simulink model "CM340A_AdcDiagc"
settings: Solver=FixedStepDiscrete  SolverMode=SingleTasking  StartTime=0.0  StopTime=1  FixedStep=0.002  RelTol=1e-3
values from neighbouring files (symbols this model uses):
  Adc0Diagc = DataDict.NTC    [CM340A_AdcDiagc_DataDict.m]
  Adc1Diagc = DataDict.NTC    [CM340A_AdcDiagc_DataDict.m]
  ADCDIAG0REFVOLT_VOLT_F32 = DataDict.Constant    [CM340A_AdcDiagc_DataDict.m]
  ADCDIAG2REFVOLT_VOLT_F32 = DataDict.Constant    [CM340A_AdcDiagc_DataDict.m]
  ADCDIAG4REFVOLT_VOLT_F32 = DataDict.Constant    [CM340A_AdcDiagc_DataDict.m]
  AdcDiagcNtc0x032FailStep = DataDict.Calibration    [CM340A_AdcDiagc_DataDict.m]
  AdcDiagcNtc0x032PassStep = DataDict.Calibration    [CM340A_AdcDiagc_DataDict.m]
  AdcDiagcNtc0x033FailStep = DataDict.Calibration    [CM340A_AdcDiagc_DataDict.m]
  AdcDiagcNtc0x033PassStep = DataDict.Calibration    [CM340A_AdcDiagc_DataDict.m]
  AdcDiagcSt = DataDict.PIM    [CM340A_AdcDiagc_DataDict.m]
  ADCDIAGPARFLTPRM_CNT_U08 = DataDict.Constant    [CM340A_AdcDiagc_DataDict.m]
  ADCDIAGSCANGROUP2REFFLTPRM_CNT_U08 = DataDict.Constant    [CM340A_AdcDiagc_DataDict.m]
  ADCDIAGSCANGROUP3REFFLTPRM_CNT_U08 = DataDict.Constant    [CM340A_AdcDiagc_DataDict.m]
  ADCDIAGSCANGROUPENDREFVOLT_VOLT_F32 = DataDict.Constant    [CM340A_AdcDiagc_DataDict.m]
  ADCDIAGSCANGROUPSTRTREFVOLT_VOLT_F32 = DataDict.Constant    [CM340A_AdcDiagc_DataDict.m]
  ADCDNECRPARERRCLR_CNT_U08 = DataDict.Constant    [CM340A_AdcDiagc_DataDict.m]
  ADCDNPERPARERRMASK_CNT_U08 = DataDict.Constant    [CM340A_AdcDiagc_DataDict.m]
  VIRTCH21_CNT_U08 = DataDict.Constant    [CM340A_AdcDiagc_DataDict.m]
  VIRTCH22_CNT_U08 = DataDict.Constant    [CM340A_AdcDiagc_DataDict.m]
  VIRTCH23_CNT_U08 = DataDict.Constant    [CM340A_AdcDiagc_DataDict.m]
undefined symbols (not defined in the file or in its folder): NtcSts1, sigbuilder_block, SigQlfr1
libraries: simulink x42, CM340A_AdcDiagc_Library x40
(part 1 of 4)
settings Model: RequirementInfo="{}  %GIDa_ca294f38_ed7c_4fb9_8c54_f4d56271bfc7"  ModifiedHistory=Rev 008: Updated model to Matlab 2013B, added comments to show requirement linkage
settings SolverCC: AutoInsertRateTranBlk=on  InsertRTBMode=Always
settings DataIOCC: SaveFormat=Structure
settings OptimizationCC: BlockReduction=off  InlineParams=on  ZeroExternalMemoryAtStartup=off  ZeroInternalMemoryAtStartup=off  OptimizeModelRefInitCode=on  LifeSpan=1  SimCompilerOptimization=Off
settings DebuggingCC: SignalInfNanChecking=error  SignalRangeChecking=warning  MergeDetectMultiDrivingBlocksExec=none  SolverPrmCheckMsg=error  InheritedTsInSrcMsg=error  DiscreteInheritContinuousMsg=error  SingleTaskRateTransMsg=error  TasksWithSamePriorityMsg=error  SigSpecEnsureSampleTimeMsg=error  CheckMatrixSingularityMsg=error  ParameterUnderflowMsg=error  ParameterPrecisionLossMsg=error  ParameterTunabilityLossMsg=error  FixptConstUnderflowMsg=warning  FixptConstOverflowMsg=warning  VectorMatrixConversionMsg=error  FcnCallInpInsideContextMsg=EnableAllAsError  SignalLabelMismatchMsg=error  UnconnectedInputMsg=error  UnconnectedOutputMsg=error  UnconnectedLineMsg=error  SFcnCompatibilityMsg=error  FrameProcessingCompatibilityMsg=warning  UniqueDataStoreMsg=warning  BusObjectLabelMismatch=error  RootOutportRequireBusObject=error  AssertControl=DisableAll  ModelReferenceIOMsg=error  ModelReferenceVersionMismatchMessage=warning  ModelReferenceIOMismatchMessage=error  ModelReferenceCSMismatchMessage=warning  ModelReferenceDataLoggingMessage=error  StateNameClashWarn=warning  StrictBusMsg=ErrorOnBusTreatedAsVector  NonBusSignalsTreatedAsBus=error  SFInvalidInputDataAccessInChartInitDiag=error  SFTransitionOutsideNaturalParentDiag=error  SFUnconditionalTransitionShadowingDiag=error  SFUndirectedBroadcastEventsDiag=error
settings HardwareCC: ProdBitPerPointer=32  ProdLargestAtomicFloat=None  ProdIntDivRoundTo=Undefined  ProdEndianess=Unspecified  ProdWordSize=32  ProdHWDeviceType=32-bit Generic
settings ModelReferenceCC: ModelReferenceNumInstancesAllowed=Single  PropagateSignalLabelsOutOfModel=off
settings SFSimCC: SimUseLocalCustomCode=off
settings RTWCC: SystemTargetFile=autosar.tlc  GenCodeOnly=on  TemplateMakefile=ert_default_tmf  Description=AUTOSAR  GenerateReport=on  ProcessScript=autosar_make_rtw_hook  RTWUseLocalCustomCode=off  LaunchReport=on  RTWCompilerOptimization=Off
settings CodeAppCC: GenerateComments=off  IgnoreCustomStorageClasses=off  CustomSymbolStrType=$N$R$M  CustomSymbolStrBlkIO=$N$M  SimulinkBlockComments=off
settings STFCustomTargetCC: CodeReplacementLibrary=ANSI_C  ParMdlRefBuildCompliant=on  CompOptLevelCompliant=on  IncludeMdlTerminateFcn=off  CombineOutputUpdateFcns=on  SuppressErrorStatus=on  ERTFirstTimeCompliant=on  ERTCustomFileBanners=on  SupportNonFinite=off  SupportComplex=off  SupportContinuousTime=off  SupportNonInlinedSFcns=off  MATLABClassNameForMDSCustomization=Simulink.SoftwareTarget.ERTCustomization  AutosarCompliant=on  GRTInterface=off  SystemTargetFile=autosar.tlc
settings ERTTargetCC: CodeReplacementLibrary=ANSI_C  MultiwordLength=2048  ConcurrentExecutionCompliant=off  IncludeMdlTerminateFcn=off  SuppressErrorStatus=on  SupportNonFinite=off  SupportComplex=off  ModelStepFunctionPrototypeControlCompliant=off  CPPClassGenCompliant=off  AutosarCompliant=on  InlinedParameterPlacement=NonHierarchical  ERTCustomFileTemplate=example_file_process.tlc  ConvertIfToSwitch=off  SuppressUnreachableDefaultCases=off  EnableUserReplacementTypes=on

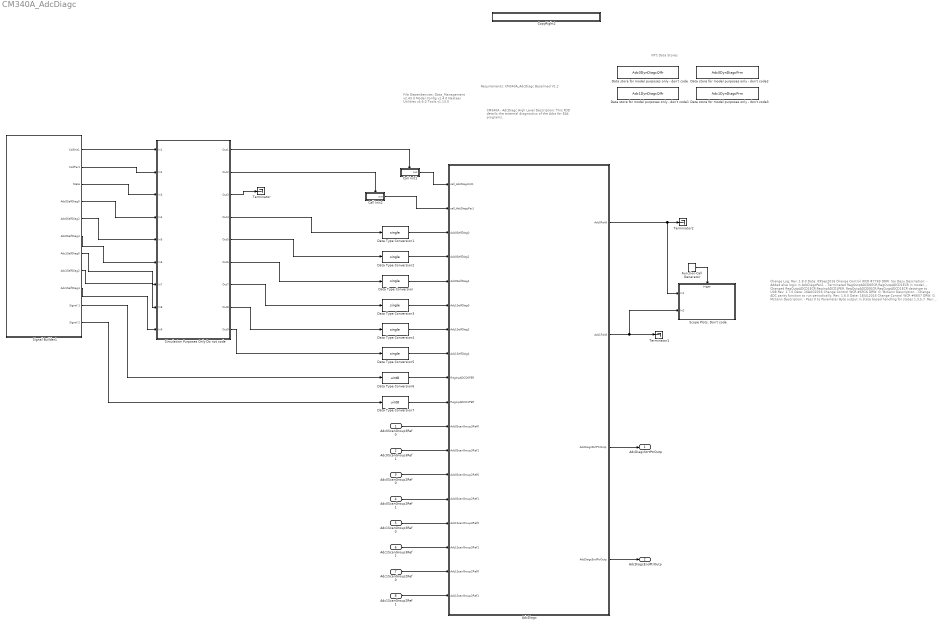
== system CM340A_AdcDiagc ==
  note: NTC Data Stores
  note: CM340A - AdcDiagc
      |
      | High Level Description:
      | This FDD details the external diagnostics of the Adcs for
      | EA4 programs.
  note: Change Log:
      |
      | Rev: 1.8.0
      | Date: 09Sep2016
      | Change Control WCR #7769
      | DRW: Sai Desu
      | Description:
      | - Added else logic in AdcDiagcPer2.
      | - Terminated RegOutpADCD0ECR,RegOutpADCD1ECR in model.
      | - Changed RegOutpADCD1ECR,RegInpADCD1PER, RegOutpADCD0ECR,RegOutpADCD1ECR datatype to U08
      |
      | Rev: 1.7.0
      | Date: 16AUG2016
      | Change Control WCR #6916
      | DRW: G. McCann
      | Description:
      | - Change ADC parity function to run periodically.
      |
      | Rev: 1.6.0
      | Date: 18JUL2016
      | Change Control WCR #6607
      | DRW: G. McCann
      | Description:
      | - Pass 0 to Parameter Byte output in state based handling for states 1,3,5,7.
      |
      | Rev: 1.5.0
      | Date: 15JUL2016
      | Change Control WCR #6588
      | DRW: G. McCann
      | Description:
      | - Change the pass and fail steps for NTCs 0x032 & 0x033 to calibrations instead of config params
      | - Change sequence of state handling in AdcDiagcPer1.  State update should happen last.
      |
      | Rev: 1.4.0
      | Date: 29JUN2016
      | Change Control WCR #6465
      | DRW: G. McCann
      | Description:
      | - Replaced stateflow with equivalent simulink blocks
      | - Requirements linkage added on new blocks
      | - Per1 Adc Diagc Pointer block executes state 6 handling for all cases where Adc Diag State != 0, 2 or 4.  Added
      |   elseif condition for handling of state 6.
      | - Same block needs to send StrtPtr and EndPtr to PIM to hold values between states 0,2,4,6
      | - The StrPtr and EndPtr PIMs should be read to update the outputs from the Adc Daigc Pointer block in Per1.
      |
      | Rev: 1.3.0
      | Date: 22JUN2016
      | Change Control WCR #6418
      | DRW: G. McCann
      | Description:
      | - Remove 'MotCtrl' prefix from I/O not connected to motor control ISR
      |
      | Rev: 1.2.0
      | Date: 07JUN2016
      | Change Control WCR #5774
      | DRW: G. McCann
      | Description:
      | - Change diagnostic parameters on AdcFltCntSt datastores for MIL testing
      | - Change register utilized for parity error check from APDPERRST to ADCDnPER
      | - Change register utilized for parity error clear from APDPERRSTC to ADCDnECR
      | - Add 4 outputs for ADCn start and end pointers (2 per ADC unit).  This change also
      |   eliminates Adc0CfgAndUseAdc0ScanGroup1Cfg and Adc1CfgAndUseAdc1ScanGroup1Cfg
      |   server functions utilized in CM300A and CM320A
      | - Add diagnostics for ADC reference read at the beginning and end of scan groups 2 & 3.  Utilize NTC
      |   Parameter bits 5&6 to accomplish this.
      |
      | Rev: 1.1.0
      | Date: 19MAR2016
      | Change Control WCR #4633,EA4#4637, EA4#4823
      | DRW: Praveen, Muragesh (KPIT)
      | Description:
      | - As per Anomaly CR EA4#3686, the Input Voltage ~= 0  condtion has been changed with
      |  Input Voltage greater than ARCHGLBPRM_FLOATZEROTHD_ULS_F32 in the CM340A_AdcDiagc_Library's
      |  zero check subsystem. ARCHGLBPRM_FLOATZEROTHD_ULS_F32 variable is defined in the .m file.
      |
      | -As per Anomaly CR EA4#3836, SetAdc0ParFlt,SetAdc1ParFlt server runnables have been merged to "SetAdcParFlt".
      | -New inputs 'RegInpAPDPERRST_ADCTL00', 'RegInpAPDPERRST_ADCTL10'
      |  and outputs 'RegOutpAPDPERRSTC_ADCTL00', 'RegOutpAPDPERRSTC_ADCTL10'
      |  and logic related to these has been added
      |
      | - As per Anomaly CR  EA4#4188, fault determination logic has been updated.
      |  8-new PIMs have been created to store fault accumulation avalue in each state for ADC0 and ADC1
      |
      | Rev: 1.0.0
      | Date: 23JAN2014
      | Change Control #: EA4#3400
      | DRW: J. Erlenbeck
      | Description:
      | - Initial Release
      |
      |
      |
      | All changes are highlighted in the red color.
  note: File Dependencies:
      | Data_Management v2.43.0
      | Model Config v1.4.0
      | Nexteer Utilities v4.6.0
      | Tools v1.13.0
  note: Requirements: CM340A_AdcDiagc Baselined V1.2
  Adc0ScanGroup3Ref0 : Inport  RequirementInfo={} %GIDa_49e55e19_ff85_4f6f_a90d_a9dcc2c0ea53
  Adc0ScanGroup3Ref1 : Inport  RequirementInfo={} %GIDa_7dd4fc61_e042_4709_b04f_f275e4d72336  Port=2
  Adc0ScanGroup2Ref0 : Inport  RequirementInfo={} %GIDa_573b7f90_76d7_4d20_8207_3d2b14b10f99  Port=3
  Adc0ScanGroup2Ref1 : Inport  RequirementInfo={} %GIDa_870086a7_d427_43e7_93f7_4a95a875be04  Port=4
  Adc1ScanGroup3Ref0 : Inport  RequirementInfo={} %GIDa_fc4d583e_0d62_4e8f_9497_a2b62302b28b  Port=5
  Adc1ScanGroup3Ref1 : Inport  RequirementInfo={} %GIDa_cad8a16f_cb5f_4c8b_be64_16977f5e4cb9  Port=6
  Adc1ScanGroup2Ref0 : Inport  RequirementInfo={} %GIDa_08b78cad_66ed_443e_a656_dce61b3506e6  Port=7
  Adc1ScanGroup2Ref1 : Inport  RequirementInfo={} %GIDa_f0961ddb_08f8_4c0a_9e27_4a6e0e526bc0  Port=8
  AdcDiagc : Subsystem
  Call Init1 : Subsystem  TreatAsAtomicUnit=on
  Call Init2 : Subsystem  TreatAsAtomicUnit=on
  CopyRight2 : Subsystem  Description=|  mask(Copyright Information){none=on}
      | Copyright info block.                                               
      |                                                                     
      | Place copyright information at the top of every subsystem in design.
      mask prompts: none "No parameters"
      mask help: Place copyright information at the top of every subsystem in design.
      mask Display:
      | NxtrConf = 'Nexteer Confidential';
      | 
      | sys = bdroot; %handle for the current model ("system")
      | first = get_param(sys,'Created');
      | first = first(end-3:end);  %year is last four digits
      | 
      | last = get_param(sys,'LastModifiedDate');
      | if isempty(last)
      |     last = datestr(now,'yyyy');
      | else
      |     last = last(end-3:end);
      | end
      | 
      | if strcmp(first,last)
      |     fprintf('%s -- Copyright %s Nexteer',NxtrConf,first)
      | else
      |     fprintf('%s -- %s%s- %s Nexteer',NxtrConf,char(169),first,last)
      | end
  Data Type Conversion{,1..5} (6 alike) : DataTypeConversion  OutDataTypeStr=single
  Data Type Conversion6 : DataTypeConversion  OutDataTypeStr=uint8
  Data Type Conversion7 : DataTypeConversion  OutDataTypeStr=uint8
  Data store for model purposes only - don't code : DataStoreMemory  DataStoreName=Adc0DynDiagcQlfr
  Data store for model purposes only - don't code1 : DataStoreMemory  DataStoreName=Adc1DynDiagcQlfr
  Data store for model purposes only - don't code2 : DataStoreMemory  DataStoreName=Adc0DynDiagcPrm
  Data store for model purposes only - don't code3 : DataStoreMemory  DataStoreName=Adc1DynDiagcPrm
  Function-Call Generator : simulink/Ports & Subsystems/Function-Call Generator  sample_time=0.002  numberOfIterations=1
  "Scope Plots, Don't code" : Subsystem  TreatAsAtomicUnit=on
  Signal Builder1 : Subsystem  Tag=STV Subsys  LoadFcn=sigbuilder_block('load');  StartFcn=sigbuilder_block('start');  StopFcn=sigbuilder_block('stop');  ClipboardFcn=sigbuilder_block('clipboard');  mask(Sigbuilder block){}
      mask help: Simulink:masks:SigbuilderBlock_MD
      mask init:
      | if ~strcmp(get_param(bdroot(gcbh),'SimulationStatus'),'stopped') tuvar = sigbuilder_block('maskInit'); end
      settings: CopyFcn=sigbuilder_block('copy');  DeleteFcn=sigbuilder_block('delete');  ModelCloseFcn=sigbuilder_block('modelClose');  PreSaveFcn=sigbuilder_block('preSave');  PauseFcn=sigbuilder_block('pause');  ContinueFcn=sigbuilder_block('continue');  NameChangeFcn=sigbuilder_block('namechange');  OpenFcn=sigbuilder_block('open',[88.5 252.75 870.75 494.25 ]);  CloseFcn=sigbuilder_block('close');
      mask Display: plot(0, 0, 100, 100,[2, 2, 32, 32, 2], [68, 8, 8, 68, 68],[32, 2], [38, 38], [32, 19, 2],[53, 60, 44], [32, 17, 17, 2],[16, 16, 31, 31]);txt = getActiveGroup(gcbh);text(2, 100, txt,'verticalAlignment', 'top');
  Simulation Purposes Only Do not code : Subsystem  TreatAsAtomicUnit=on
  Terminator : Terminator
  Terminator1 : Terminator
  Terminator2 : Terminator
  AdcDiagcStrtPtrOutp : Outport
  AdcDiagcEndPtrOutp : Outport  Port=2
  wires:
  Call Init1/1(out) -> AdcDiagc/1(call_AdcDiagcInit1)
  Call Init2/1(out) -> AdcDiagc/2(call_AdcDiagcPer1)
  Data Type Conversion1/1 -> AdcDiagc/3(Adc0SelfDiag0)
  Data Type Conversion2/1 -> AdcDiagc/4(Adc0SelfDiag2)
  Data Type Conversion/1 -> AdcDiagc/5(Adc0SelfDiag4)
  Simulation Purposes Only Do not code/1(Out1) -> Call Init1/Enable
  Simulation Purposes Only Do not code/2(Out2) -> Call Init2/Enable
  Simulation Purposes Only Do not code/4(Out4) -> Data Type Conversion1/1
  Simulation Purposes Only Do not code/5(Out5) -> Data Type Conversion2/1
  Simulation Purposes Only Do not code/6(Out6) -> Data Type Conversion/1
  Simulation Purposes Only Do not code/3(Out3) -> Terminator/1
  Simulation Purposes Only Do not code/7(Out7) -> Data Type Conversion3/1
  Simulation Purposes Only Do not code/8(Out8) -> Data Type Conversion4/1
  Simulation Purposes Only Do not code/9(Out9) -> Data Type Conversion5/1
  Data Type Conversion3/1 -> AdcDiagc/6(Adc1SelfDiag0)
  Data Type Conversion4/1 -> AdcDiagc/7(Adc1SelfDiag2)
  Data Type Conversion5/1 -> AdcDiagc/8(Adc1SelfDiag4)
  AdcDiagc/1(Adc0Faild) -> Terminator2/1, "Scope Plots, Don't code"/1(In1)
  AdcDiagc/2(Adc1Faild) -> Terminator1/1, "Scope Plots, Don't code"/2(In2)
  Signal Builder1/2(CallPer1) -> Simulation Purposes Only Do not code/2(In2)
  Signal Builder1/3(State) -> Simulation Purposes Only Do not code/3(In3)
  Signal Builder1/1(CallInit1) -> Simulation Purposes Only Do not code/1(In1)
  Signal Builder1/8(Adc1SelfDiag2) -> Simulation Purposes Only Do not code/8(In8)
  Signal Builder1/5(Adc0SelfDiag2) -> Simulation Purposes Only Do not code/5(In5)
  Signal Builder1/7(Adc1SelfDiag0) -> Simulation Purposes Only Do not code/7(In7)
  Signal Builder1/4(Adc0SelfDiag0) -> Simulation Purposes Only Do not code/4(In4)
  Signal Builder1/6(Adc0SelfDiag4) -> Simulation Purposes Only Do not code/6(In6)
  Signal Builder1/9(Adc1SelfDiag4) -> Simulation Purposes Only Do not code/9(In9)
  Data Type Conversion6/1 -> AdcDiagc/9(RegInpADCD0PER)
  Data Type Conversion7/1 -> AdcDiagc/10(RegInpADCD1PER)
  AdcDiagc/3(AdcDiagcStrtPtrOutp) -> AdcDiagcStrtPtrOutp/1
  AdcDiagc/4(AdcDiagcEndPtrOutp) -> AdcDiagcEndPtrOutp/1
  Adc0ScanGroup3Ref0/1 -> AdcDiagc/11(Adc0ScanGroup3Ref0)
  Adc0ScanGroup3Ref1/1 -> AdcDiagc/12(Adc0ScanGroup3Ref1)
  Adc0ScanGroup2Ref0/1 -> AdcDiagc/13(Adc0ScanGroup2Ref0)
  Adc0ScanGroup2Ref1/1 -> AdcDiagc/14(Adc0ScanGroup2Ref1)
  Adc1ScanGroup3Ref0/1 -> AdcDiagc/15(Adc1ScanGroup3Ref0)
  Adc1ScanGroup3Ref1/1 -> AdcDiagc/16(Adc1ScanGroup3Ref1)
  Adc1ScanGroup2Ref0/1 -> AdcDiagc/17(Adc1ScanGroup2Ref0)
  Adc1ScanGroup2Ref1/1 -> AdcDiagc/18(Adc1ScanGroup2Ref1)
  Function-Call Generator/1 -> "Scope Plots, Don't code"/Trigger
  Signal Builder1/10(Signal 1) -> Data Type Conversion6/1
  Signal Builder1/11(Signal 2) -> Data Type Conversion7/1

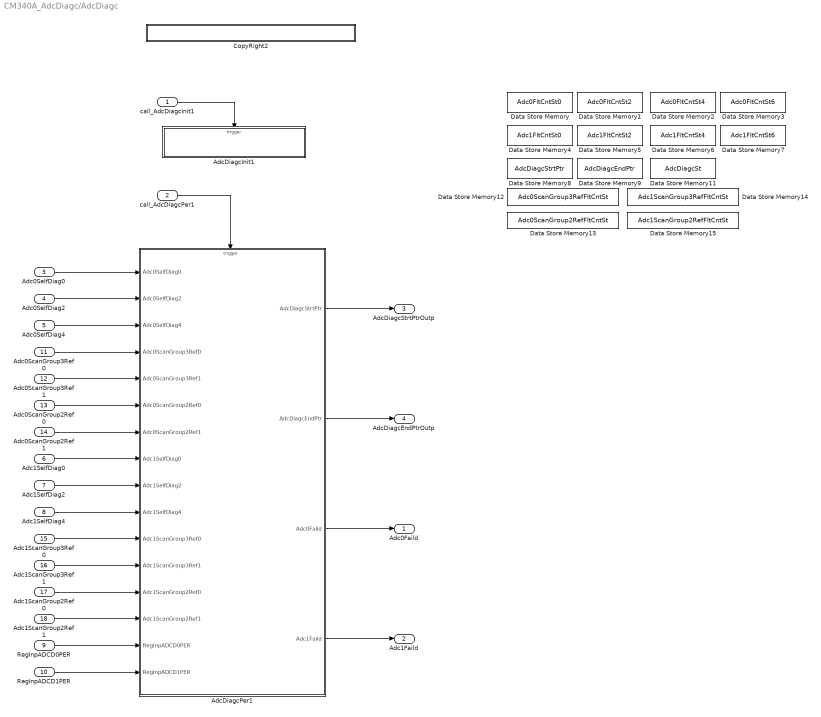
== system CM340A_AdcDiagc/AdcDiagc ==
  call_AdcDiagcInit1 : Inport  RequirementInfo={} %GIDa_18b4b7a7_d8ff_42fd_afd9_8fbc558fb7ae
  call_AdcDiagcPer1 : Inport  RequirementInfo={} %GIDa_8c56c68f_1996_47ee_bda4_35b4dc112bcf  Port=2
  Adc0SelfDiag0 : Inport  RequirementInfo={} %GIDa_768985a4_e900_425c_ae1d_47338650e664  Port=3
  Adc0SelfDiag2 : Inport  RequirementInfo={} %GIDa_3fc10c39_7c74_41d4_a880_daee12f7febc  Port=4
  Adc0SelfDiag4 : Inport  RequirementInfo={} %GIDa_be7414d0_49f3_45cb_bfb1_3ce36dce7edf  Port=5
  Adc1SelfDiag0 : Inport  RequirementInfo={} %GIDa_0acfad8b_9c66_4bcf_95d2_4b0e54aa7e17  Port=6
  Adc1SelfDiag2 : Inport  RequirementInfo={} %GIDa_b99c857a_5fe3_43c9_8cf6_48a3f2428904  Port=7
  Adc1SelfDiag4 : Inport  RequirementInfo={} %GIDa_bb8ad16f_1b31_4872_b9ab_2443b8d4b36b  Port=8
  RegInpADCD0PER : Inport  RequirementInfo={} %GIDa_1c4b2026_055f_43fd_ac9a_1a1cfd812325  Port=9
  RegInpADCD1PER : Inport  RequirementInfo={} %GIDa_ff327575_5ab9_43e4_9182_a2fefb3f953b  Port=10
  Adc0ScanGroup3Ref0 : Inport  RequirementInfo={} %GIDa_bab94f49_6424_4c49_888e_5ff6776a5db3  Port=11
  Adc0ScanGroup3Ref1 : Inport  RequirementInfo={} %GIDa_98f92e48_b093_40f2_8328_2158e7be4df2  Port=12
  Adc0ScanGroup2Ref0 : Inport  RequirementInfo={} %GIDa_ab2ebf3d_54de_4695_942c_c5c65492a51c  Port=13
  Adc0ScanGroup2Ref1 : Inport  RequirementInfo={} %GIDa_8b71ec07_3ef8_4676_a6fa_bdb7f3897266  Port=14
  Adc1ScanGroup3Ref0 : Inport  RequirementInfo={} %GIDa_572c4384_6519_48a1_aa24_069bc074be5f  Port=15
  Adc1ScanGroup3Ref1 : Inport  RequirementInfo={} %GIDa_259d8fd0_61d2_4bba_b7a5_11056a435558  Port=16
  Adc1ScanGroup2Ref0 : Inport  RequirementInfo={} %GIDa_18152ad2_e8f7_4af5_a23a_ab069d03dc39  Port=17
  Adc1ScanGroup2Ref1 : Inport  RequirementInfo={} %GIDa_93789243_a541_499f_9474_e657f20cd06a  Port=18
  AdcDiagcInit1 : Subsystem
  AdcDiagcPer1 : Subsystem  RequirementInfo="{'linktype_rmi_doors' '000079f2 (/ESG Group/FDD Module Requirements/EA4 Specific/CM340A_AdcDiagc)' '#CM340A_16' 'true' 'REQ:  CM340A_16' '' ; 'linktype_rmi_doors' '000079f2 (/ESG Group/FDD Module Requirements/EA4 Specific/CM340A_AdcDiagc)' '#CM340A_70' 'true' 'REQ:  CM340A_70' '' ; 'linktype_rmi_doors' '000079f2 (/ESG Group/FDD Module Requirements/EA4 Specific/CM340A_AdcDiagc)' '#CM340A_204' 'true' 'REQ:  CM340A_204' '' } %GIDa_212d137a_62a0_40b8_86f5_bba5fab12a7f"  TreatAsAtomicUnit=on
  CopyRight2 : Subsystem  Description=|  mask(Copyright Information){none=on}
      | Copyright info block.                                               
      |                                                                     
      | Place copyright information at the top of every subsystem in design.
      mask prompts: none "No parameters"
      mask help: Place copyright information at the top of every subsystem in design.
      mask Display:
      | NxtrConf = 'Nexteer Confidential';
      | 
      | sys = bdroot; %handle for the current model ("system")
      | first = get_param(sys,'Created');
      | first = first(end-3:end);  %year is last four digits
      | 
      | last = get_param(sys,'LastModifiedDate');
      | if isempty(last)
      |     last = datestr(now,'yyyy');
      | else
      |     last = last(end-3:end);
      | end
      | 
      | if strcmp(first,last)
      |     fprintf('%s -- Copyright %s Nexteer',NxtrConf,first)
      | else
      |     fprintf('%s -- %s%s- %s Nexteer',NxtrConf,char(169),first,last)
      | end
  Data Store Memory : DataStoreMemory  DataStoreName=Adc0FltCntSt0  StateMustResolveToSignalObject=on
  Data Store Memory1 : DataStoreMemory  DataStoreName=Adc0FltCntSt2  StateMustResolveToSignalObject=on
  Data Store Memory11 : DataStoreMemory  DataStoreName=AdcDiagcSt  StateMustResolveToSignalObject=on
  Data Store Memory12 : DataStoreMemory  DataStoreName=Adc0ScanGroup3RefFltCntSt  StateMustResolveToSignalObject=on
  Data Store Memory13 : DataStoreMemory  DataStoreName=Adc0ScanGroup2RefFltCntSt  StateMustResolveToSignalObject=on
  Data Store Memory14 : DataStoreMemory  DataStoreName=Adc1ScanGroup3RefFltCntSt  StateMustResolveToSignalObject=on
  Data Store Memory15 : DataStoreMemory  DataStoreName=Adc1ScanGroup2RefFltCntSt  StateMustResolveToSignalObject=on
  Data Store Memory2 : DataStoreMemory  DataStoreName=Adc0FltCntSt4  StateMustResolveToSignalObject=on
  Data Store Memory3 : DataStoreMemory  DataStoreName=Adc0FltCntSt6  StateMustResolveToSignalObject=on
  Data Store Memory4 : DataStoreMemory  DataStoreName=Adc1FltCntSt0  StateMustResolveToSignalObject=on
  Data Store Memory5 : DataStoreMemory  DataStoreName=Adc1FltCntSt2  StateMustResolveToSignalObject=on
  Data Store Memory6 : DataStoreMemory  DataStoreName=Adc1FltCntSt4  StateMustResolveToSignalObject=on
  Data Store Memory7 : DataStoreMemory  DataStoreName=Adc1FltCntSt6  StateMustResolveToSignalObject=on
  Data Store Memory8 : DataStoreMemory  DataStoreName=AdcDiagcStrtPtr  StateMustResolveToSignalObject=on
  Data Store Memory9 : DataStoreMemory  DataStoreName=AdcDiagcEndPtr  StateMustResolveToSignalObject=on
  Adc0Faild : Outport
  Adc1Faild : Outport  Port=2
  AdcDiagcStrtPtrOutp : Outport  Port=3
  AdcDiagcEndPtrOutp : Outport  Port=4
  wires:
  call_AdcDiagcInit1/1 -> AdcDiagcInit1/Trigger
  call_AdcDiagcPer1/1 -> AdcDiagcPer1/Trigger
  Adc0SelfDiag0/1 -> AdcDiagcPer1/1(Adc0SelfDiag0)
  Adc0SelfDiag2/1 -> AdcDiagcPer1/2(Adc0SelfDiag2)
  Adc0SelfDiag4/1 -> AdcDiagcPer1/3(Adc0SelfDiag4)
  Adc1SelfDiag0/1 -> AdcDiagcPer1/8(Adc1SelfDiag0)
  Adc1SelfDiag2/1 -> AdcDiagcPer1/9(Adc1SelfDiag2)
  Adc1SelfDiag4/1 -> AdcDiagcPer1/10(Adc1SelfDiag4)
  Adc0ScanGroup3Ref0/1 -> AdcDiagcPer1/4(Adc0ScanGroup3Ref0)
  Adc0ScanGroup3Ref1/1 -> AdcDiagcPer1/5(Adc0ScanGroup3Ref1)
  Adc0ScanGroup2Ref0/1 -> AdcDiagcPer1/6(Adc0ScanGroup2Ref0)
  Adc0ScanGroup2Ref1/1 -> AdcDiagcPer1/7(Adc0ScanGroup2Ref1)
  Adc1ScanGroup3Ref0/1 -> AdcDiagcPer1/11(Adc1ScanGroup3Ref0)
  Adc1ScanGroup3Ref1/1 -> AdcDiagcPer1/12(Adc1ScanGroup3Ref1)
  Adc1ScanGroup2Ref0/1 -> AdcDiagcPer1/13(Adc1ScanGroup2Ref0)
  Adc1ScanGroup2Ref1/1 -> AdcDiagcPer1/14(Adc1ScanGroup2Ref1)
  AdcDiagcPer1/1(AdcDiagcStrtPtr) -> AdcDiagcStrtPtrOutp/1
  AdcDiagcPer1/2(AdcDiagcEndPtr) -> AdcDiagcEndPtrOutp/1
  RegInpADCD0PER/1 -> AdcDiagcPer1/15(RegInpADCD0PER)
  RegInpADCD1PER/1 -> AdcDiagcPer1/16(RegInpADCD1PER)
  AdcDiagcPer1/3(Adc0Faild) -> Adc0Faild/1
  AdcDiagcPer1/4(Adc1Faild) -> Adc1Faild/1

== system CM340A_AdcDiagc/Call Init1 ==
  Enable : EnablePort
  Function Call Trigger : simulink/Ports & Subsystems/Function-Call Generator  RequirementInfo={} %GIDa_ff755a2e_49d1_45f7_8591_3ce0ef475338  sample_time=0.002  numberOfIterations=1
  out : Outport
  wires:
  Function Call Trigger/1 -> out/1

== system CM340A_AdcDiagc/Call Init2 ==
  Enable : EnablePort
  Function Call Trigger : simulink/Ports & Subsystems/Function-Call Generator  RequirementInfo={} %GIDa_6dd05ab1_f91b_4d7a_a0ec_1170d213fa7b  sample_time=0.002  numberOfIterations=1
  out : Outport
  wires:
  Function Call Trigger/1 -> out/1

== system CM340A_AdcDiagc/CopyRight2 ==

== system CM340A_AdcDiagc/Scope Plots, Don't code ==
  In1 : Inport
  In2 : Inport  Port=2
  function : TriggerPort  TriggerType=function-call
  Data Store Read : DataStoreRead  DataStoreName=Adc0DynDiagcPrm
  Data Store Read1 : DataStoreRead  DataStoreName=Adc1DynDiagcPrm
  Display : Display
  Display1 : Display
  Scope : Scope  NumInputPorts=4
      settings: YMin=-5~-5~-5~-5  YMax=5~5~5~5
  wires:
  Data Store Read/1 -> Display/1, Scope/2
  Data Store Read1/1 -> Display1/1, Scope/4
  In1/1 -> Scope/1
  In2/1 -> Scope/3

== system CM340A_AdcDiagc/Signal Builder1 ==
  Demux : Demux  Tag=STV Demux  Outputs=11
  FromWs : FromWorkspace  Tag=STV FromWs  VariableName=tuvar  SampleTime=0
  CallInit1 : Outport
  CallPer1 : Outport  Tag=STV Outport  Port=2
  State : Outport  Tag=STV Outport  Port=3
  Adc0SelfDiag0 : Outport  Tag=STV Outport  Port=4
  Adc0SelfDiag2 : Outport  Tag=STV Outport  Port=5
  Adc0SelfDiag4 : Outport  Tag=STV Outport  Port=6
  Adc1SelfDiag0 : Outport  Tag=STV Outport  Port=7
  Adc1SelfDiag2 : Outport  Tag=STV Outport  Port=8
  Adc1SelfDiag4 : Outport  Tag=STV Outport  Port=9
  Signal 1 : Outport  Tag=STV Outport  Port=10
  Signal 2 : Outport  Tag=STV Outport  Port=11
  wires:
  Demux/1 -> CallInit1/1
  FromWs/1 -> Demux/1
  Demux/2 -> CallPer1/1
  Demux/3 -> State/1
  Demux/4 -> Adc0SelfDiag0/1
  Demux/5 -> Adc0SelfDiag2/1
  Demux/6 -> Adc0SelfDiag4/1
  Demux/7 -> Adc1SelfDiag0/1
  Demux/8 -> Adc1SelfDiag2/1
  Demux/9 -> Adc1SelfDiag4/1
  Demux/10 -> Signal 1/1
  Demux/11 -> Signal 2/1

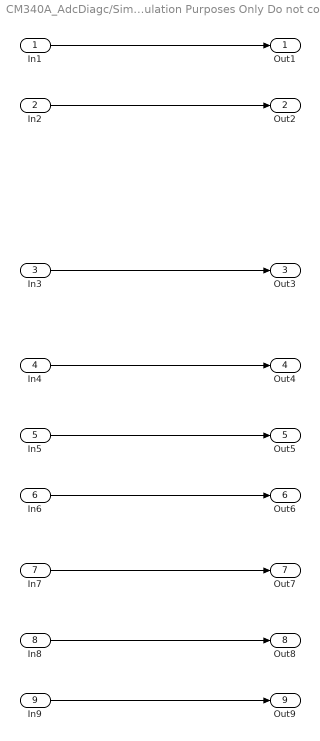
== system CM340A_AdcDiagc/Simulation Purposes Only Do not code ==
  In1 : Inport
  In2 : Inport  Port=2
  In3 : Inport  Port=3
  In4 : Inport  Port=4
  In5 : Inport  Port=5
  In6 : Inport  Port=6
  In7 : Inport  Port=7
  In8 : Inport  Port=8
  In9 : Inport  Port=9
  Out1 : Outport
  Out2 : Outport  Port=2
  Out3 : Outport  Port=3
  Out4 : Outport  Port=4
  Out5 : Outport  Port=5
  Out6 : Outport  Port=6
  Out7 : Outport  Port=7
  Out8 : Outport  Port=8
  Out9 : Outport  Port=9
  wires:
  In1/1 -> Out1/1
  In2/1 -> Out2/1
  In3/1 -> Out3/1
  In4/1 -> Out4/1
  In5/1 -> Out5/1
  In6/1 -> Out6/1
  In7/1 -> Out7/1
  In8/1 -> Out8/1
  In9/1 -> Out9/1

== system CM340A_AdcDiagc/AdcDiagc/AdcDiagcInit1 ==
  function : TriggerPort  TriggerType=function-call
  CopyRight2 : Subsystem  Description=|  mask(Copyright Information){none=on}
      | Copyright info block.                                               
      |                                                                     
      | Place copyright information at the top of every subsystem in design.
      mask prompts: none "No parameters"
      mask help: Place copyright information at the top of every subsystem in design.
      mask Display:
      | NxtrConf = 'Nexteer Confidential';
      | 
      | sys = bdroot; %handle for the current model ("system")
      | first = get_param(sys,'Created');
      | first = first(end-3:end);  %year is last four digits
      | 
      | last = get_param(sys,'LastModifiedDate');
      | if isempty(last)
      |     last = datestr(now,'yyyy');
      | else
      |     last = last(end-3:end);
      | end
      | 
      | if strcmp(first,last)
      |     fprintf('%s -- Copyright %s Nexteer',NxtrConf,first)
      | else
      |     fprintf('%s -- %s%s- %s Nexteer',NxtrConf,char(169),first,last)
      | end

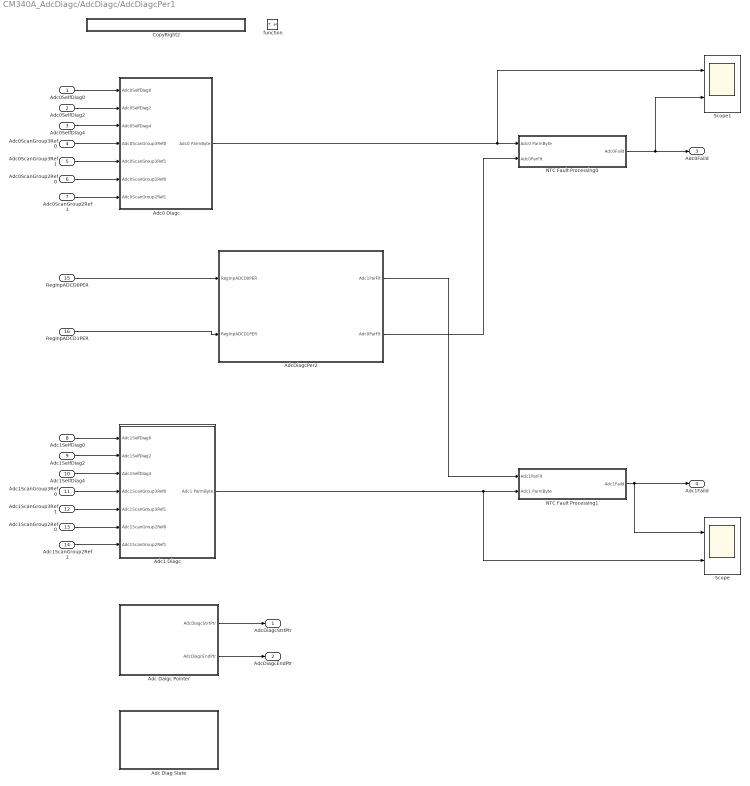
== system CM340A_AdcDiagc/AdcDiagc/AdcDiagcPer1 ==
  Adc0SelfDiag0 : Inport  RequirementInfo={} %GIDa_398af57d_66f9_4248_8190_db0e776b721c
  Adc0SelfDiag2 : Inport  RequirementInfo={} %GIDa_3797a2ee_2714_4505_8d9f_c06ba9c2410a  Port=2
  Adc0SelfDiag4 : Inport  RequirementInfo={} %GIDa_1ba69c54_a3c2_4a1b_b281_43e29c60c561  Port=3
  Adc0ScanGroup3Ref0 : Inport  RequirementInfo={} %GIDa_b69125fd_1372_4953_9f1d_8e09c2ad4765  Port=4
  Adc0ScanGroup3Ref1 : Inport  RequirementInfo={} %GIDa_f2d9eb47_94c7_42c7_a565_8454874220f9  Port=5
  Adc0ScanGroup2Ref0 : Inport  RequirementInfo={} %GIDa_748996a5_f302_4c6d_9251_b06a31b520da  Port=6
  Adc0ScanGroup2Ref1 : Inport  RequirementInfo={} %GIDa_62cd2350_592e_4caf_8293_5786819e876e  Port=7
  Adc1SelfDiag0 : Inport  RequirementInfo={} %GIDa_5433d538_46b8_4710_9f51_90a1755e5365  Port=8
  Adc1SelfDiag2 : Inport  RequirementInfo={} %GIDa_cf98083c_832e_42bb_b714_4f1778ae5820  Port=9
  Adc1SelfDiag4 : Inport  RequirementInfo={} %GIDa_f0469ca3_52bb_4d75_9ba6_24b9dcc42878  Port=10
  Adc1ScanGroup3Ref0 : Inport  RequirementInfo={} %GIDa_8fb83cb2_3080_4b0a_be49_1e0ee5149889  Port=11
  Adc1ScanGroup3Ref1 : Inport  RequirementInfo={} %GIDa_9cfb09be_3cef_48c6_a43d_b09581d94508  Port=12
  Adc1ScanGroup2Ref0 : Inport  RequirementInfo={} %GIDa_19dd82f8_e08f_4772_9f75_eda53b43109c  Port=13
  Adc1ScanGroup2Ref1 : Inport  RequirementInfo={} %GIDa_5081205f_adca_4d34_ac0d_2760b9b6cbb4  Port=14
  RegInpADCD0PER : Inport  RequirementInfo={} %GIDa_f892c6be_11e8_41e7_9539_6ea24d7285ca  Port=15
  RegInpADCD1PER : Inport  RequirementInfo={} %GIDa_fb1af02a_ee48_4694_a668_6f65c74c073f  Port=16
  function : TriggerPort  TriggerType=function-call
  Adc Daigc Pointer : Subsystem  Priority=20
      settings: AttributesFormatString=Priority=%<Priority>
  Adc Diag State : Subsystem  RequirementInfo="{'linktype_rmi_doors' '000079f2 (/ESG Group/FDD Module Requirements/EA4 Specific/CM340A_AdcDiagc)' '#CM340A_194' 'true' 'REQ:  CM340A_194' '' ; 'linktype_rmi_doors' '000079f2 (/ESG Group/FDD Module Requirements/EA4 Specific/CM340A_AdcDiagc)' '#CM340A_102' 'true' 'REQ:  CM340A_102' '' ; 'linktype_rmi_doors' '000079f2 (/ESG Group/FDD Module Requirements/EA4 Specific/CM340A_AdcDiagc)' '#CM340A_112' 'true' 'REQ:  CM340A_112' '' } %GIDa_801c7126_d3ff_4755_b335_51df2b5f807d"  Priority=40  TreatAsAtomicUnit=on
      settings: AttributesFormatString=Priority = %<Priority>
  Adc0 Diagc : Subsystem  Priority=5  TreatAsAtomicUnit=on
      settings: AttributesFormatString=Priority=%<Priority>
  Adc1 Diagc : Subsystem  Priority=10  TreatAsAtomicUnit=on
      settings: AttributesFormatString=Priority=%<Priority>
  AdcDiagcPer2 : Subsystem  RequirementInfo="{'linktype_rmi_doors' '000079f2 (/ESG Group/FDD Module Requirements/EA4 Specific/CM340A_AdcDiagc)' '#CM340A_206' 'true' 'REQ:  CM340A_206' '' } %GIDa_5b7560d5_8186_4135_8b2d_fba8c958e2d9"  Priority=0
      settings: AttributesFormatString=Priority = %<Priority>
  CopyRight2 : Subsystem  Description=|  mask(Copyright Information){none=on}
      | Copyright info block.                                               
      |                                                                     
      | Place copyright information at the top of every subsystem in design.
      mask prompts: none "No parameters"
      mask help: Place copyright information at the top of every subsystem in design.
      mask Display:
      | NxtrConf = 'Nexteer Confidential';
      | 
      | sys = bdroot; %handle for the current model ("system")
      | first = get_param(sys,'Created');
      | first = first(end-3:end);  %year is last four digits
      | 
      | last = get_param(sys,'LastModifiedDate');
      | if isempty(last)
      |     last = datestr(now,'yyyy');
      | else
      |     last = last(end-3:end);
      | end
      | 
      | if strcmp(first,last)
      |     fprintf('%s -- Copyright %s Nexteer',NxtrConf,first)
      | else
      |     fprintf('%s -- %s%s- %s Nexteer',NxtrConf,char(169),first,last)
      | end
  NTC Fault Processing0 : Subsystem  RequirementInfo="{'linktype_rmi_doors' '000079f2 (/ESG Group/FDD Module Requirements/EA4 Specific/CM340A_AdcDiagc)' '#CM340A_200' 'true' 'REQ:  CM340A_200' '' ; 'linktype_rmi_doors' '000079f2 (/ESG Group/FDD Module Requirements/EA4 Specific/CM340A_AdcDiagc)' '#CM340A_122' 'true' 'REQ:  CM340A_122' '' } %GIDa_4d05836e_001f_46e0_8cc5_082fda3c5ac5"  TreatAsAtomicUnit=on
  NTC Fault Processing1 : Subsystem  RequirementInfo="{'linktype_rmi_doors' '000079f2 (/ESG Group/FDD Module Requirements/EA4 Specific/CM340A_AdcDiagc)' '#CM340A_203' 'true' 'REQ:  CM340A_203' '' ; 'linktype_rmi_doors' '000079f2 (/ESG Group/FDD Module Requirements/EA4 Specific/CM340A_AdcDiagc)' '#CM340A_132' 'true' 'REQ:  CM340A_132' '' } %GIDa_2135f153_303a_4bc7_a24b_680511b64853"  TreatAsAtomicUnit=on
  Scope : Scope  NumInputPorts=2
      settings: YMin=-5~-5  YMax=5~5
  Scope1 : Scope  NumInputPorts=2
      settings: YMin=-5~-5  YMax=5~5  SaveName=ScopeData9
  AdcDiagcStrtPtr : Outport
  AdcDiagcEndPtr : Outport  Port=2
  Adc0Faild : Outport  Port=3
  Adc1Faild : Outport  Port=4
  wires:
  Adc1SelfDiag0/1 -> Adc1 Diagc/1(Adc1SelfDiag0)
  Adc1SelfDiag2/1 -> Adc1 Diagc/2(Adc1SelfDiag2)
  Adc1SelfDiag4/1 -> Adc1 Diagc/3(Adc1SelfDiag4)
  Adc0SelfDiag0/1 -> Adc0 Diagc/1(Adc0SelfDiag0)
  Adc0SelfDiag2/1 -> Adc0 Diagc/2(Adc0SelfDiag2)
  Adc0SelfDiag4/1 -> Adc0 Diagc/3(Adc0SelfDiag4)
  Adc0ScanGroup3Ref0/1 -> Adc0 Diagc/4(Adc0ScanGroup3Ref0)
  Adc0ScanGroup3Ref1/1 -> Adc0 Diagc/5(Adc0ScanGroup3Ref1)
  Adc0ScanGroup2Ref0/1 -> Adc0 Diagc/6(Adc0ScanGroup2Ref0)
  Adc0ScanGroup2Ref1/1 -> Adc0 Diagc/7(Adc0ScanGroup2Ref1)
  Adc1ScanGroup3Ref0/1 -> Adc1 Diagc/4(Adc1ScanGroup3Ref0)
  Adc1ScanGroup3Ref1/1 -> Adc1 Diagc/5(Adc1ScanGroup3Ref1)
  Adc1ScanGroup2Ref0/1 -> Adc1 Diagc/6(Adc1ScanGroup2Ref0)
  Adc1ScanGroup2Ref1/1 -> Adc1 Diagc/7(Adc1ScanGroup2Ref1)
  Adc Daigc Pointer/1(AdcDiagcStrtPtr) -> AdcDiagcStrtPtr/1
  Adc Daigc Pointer/2(AdcDiagcEndPtr) -> AdcDiagcEndPtr/1
  RegInpADCD0PER/1 -> AdcDiagcPer2/1(RegInpADCD0PER)
  RegInpADCD1PER/1 -> AdcDiagcPer2/2(RegInpADCD1PER)
  NTC Fault Processing0/1(Adc0Faild) -> Scope1/2, Adc0Faild/1
  Adc0 Diagc/1(Adc0 ParmByte) -> Scope1/1, NTC Fault Processing0/1(Adc0 ParmByte)
  NTC Fault Processing1/1(Adc1Faild) -> Scope/1, Adc1Faild/1
  Adc1 Diagc/1(Adc1 ParmByte) -> Scope/2, NTC Fault Processing1/2(Adc1 ParmByte)
  AdcDiagcPer2/2(Adc0ParFlt) -> NTC Fault Processing0/2(Adc0ParFlt)
  AdcDiagcPer2/1(Adc1ParFlt) -> NTC Fault Processing1/1(Adc1ParFlt)

== system CM340A_AdcDiagc/AdcDiagc/CopyRight2 ==

== system CM340A_AdcDiagc/AdcDiagc/AdcDiagcInit1/CopyRight2 ==

== system CM340A_AdcDiagc/AdcDiagc/AdcDiagcPer1/Adc Daigc Pointer ==
  CopyRight2 : Subsystem  Description=|  mask(Copyright Information){none=on}
      | Copyright info block.                                               
      |                                                                     
      | Place copyright information at the top of every subsystem in design.
      mask prompts: none "No parameters"
      mask help: Place copyright information at the top of every subsystem in design.
      mask Display:
      | NxtrConf = 'Nexteer Confidential';
      | 
      | sys = bdroot; %handle for the current model ("system")
      | first = get_param(sys,'Created');
      | first = first(end-3:end);  %year is last four digits
      | 
      | last = get_param(sys,'LastModifiedDate');
      | if isempty(last)
      |     last = datestr(now,'yyyy');
      | else
      |     last = last(end-3:end);
      | end
      | 
      | if strcmp(first,last)
      |     fprintf('%s -- Copyright %s Nexteer',NxtrConf,first)
      | else
      |     fprintf('%s -- %s%s- %s Nexteer',NxtrConf,char(169),first,last)
      | end
  Data Store Read : DataStoreRead  DataStoreName=AdcDiagcSt
  Strt & End Ptr Output : Subsystem  Priority=2
      settings: AttributesFormatString=Priority = %<Priority>
  Strt & End Ptr Store : Subsystem  Priority=1
      settings: AttributesFormatString=Priority = %<Priority>
  AdcDiagcStrtPtr : Outport
  AdcDiagcEndPtr : Outport  Port=2
  wires:
  Data Store Read/1 -> Strt & End Ptr Store/1(Adc Diag State)
  Strt & End Ptr Output/1(AdcDiagcStrtPtr) -> AdcDiagcStrtPtr/1
  Strt & End Ptr Output/2(AdcDiagcEndPtr) -> AdcDiagcEndPtr/1

== system CM340A_AdcDiagc/AdcDiagc/AdcDiagcPer1/Adc Diag State ==
  note: ***********************************************
      | Note that this mechanism of
      | rolling back the state to 0 with this
      | method only works when
      | AdcDiagcSt.EngMax = 7.  If the diagnostic
      | changes this technique will have to be revisted
      | ***********************************************
  Add : Sum
  Bitwise Operator : simulink/Logic and Bit Operations/Bitwise Operator  logicop=AND  UseBitMask=off  NumInputPorts=2  BitMask=bin2dec('11011001')  BitMaskRealWorld=Stored Integer
  Constant : Constant  OutDataTypeStr=uint8
  Constant1 : Constant  Value=AdcDiagcSt.EngMax
  CopyRight2 : Subsystem  Description=|  mask(Copyright Information){none=on}
      | Copyright info block.                                               
      |                                                                     
      | Place copyright information at the top of every subsystem in design.
      mask prompts: none "No parameters"
      mask help: Place copyright information at the top of every subsystem in design.
      mask Display:
      | NxtrConf = 'Nexteer Confidential';
      | 
      | sys = bdroot; %handle for the current model ("system")
      | first = get_param(sys,'Created');
      | first = first(end-3:end);  %year is last four digits
      | 
      | last = get_param(sys,'LastModifiedDate');
      | if isempty(last)
      |     last = datestr(now,'yyyy');
      | else
      |     last = last(end-3:end);
      | end
      | 
      | if strcmp(first,last)
      |     fprintf('%s -- Copyright %s Nexteer',NxtrConf,first)
      | else
      |     fprintf('%s -- %s%s- %s Nexteer',NxtrConf,char(169),first,last)
      | end
  Data Store Read : DataStoreRead  DataStoreName=AdcDiagcSt
  Data Store Write : DataStoreWrite  DataStoreName=AdcDiagcSt
  Data Type Conversion : DataTypeConversion  OutDataTypeStr=uint8
  wires:
  Constant/1 -> Add/1
  Constant1/1 -> Data Type Conversion/1
  Add/1 -> Bitwise Operator/2
  Data Type Conversion/1 -> Bitwise Operator/1
  Data Store Read/1 -> Add/2
  Bitwise Operator/1 -> Data Store Write/1

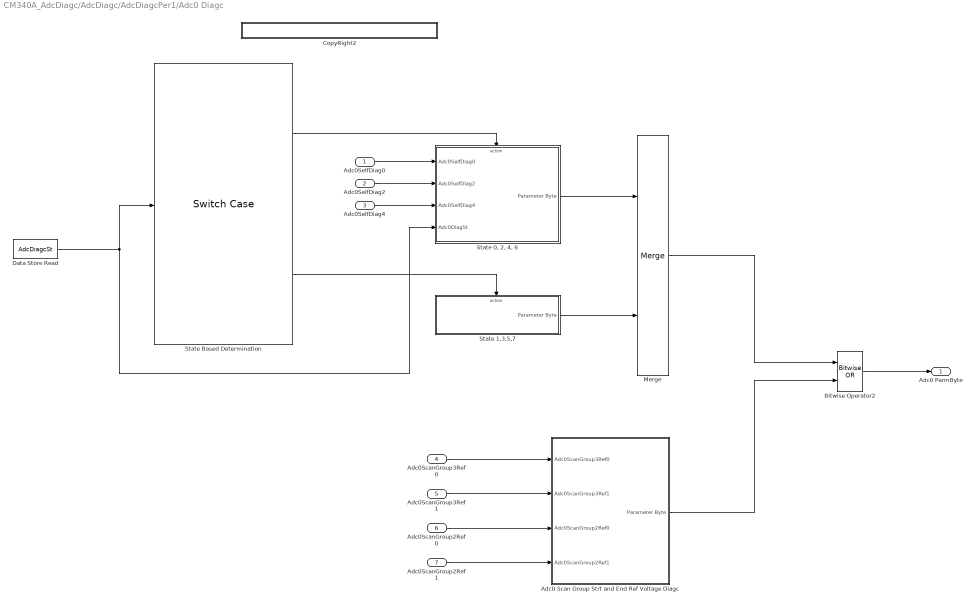
== system CM340A_AdcDiagc/AdcDiagc/AdcDiagcPer1/Adc0 Diagc ==
  Adc0SelfDiag0 : Inport  RequirementInfo={} %GIDa_8c44b7b5_be32_46ad_bd4e_9c60b23c45a8
  Adc0SelfDiag2 : Inport  RequirementInfo={} %GIDa_a296aa7a_0e47_453a_a758_f77e1172a5a6  Port=2
  Adc0SelfDiag4 : Inport  RequirementInfo={} %GIDa_a98d8dd3_9f46_4309_b7f1_a50f146190a2  Port=3
  Adc0ScanGroup3Ref0 : Inport  RequirementInfo={} %GIDa_11954da4_53ef_4f14_b015_a9bd1937ba50  Port=4
  Adc0ScanGroup3Ref1 : Inport  RequirementInfo={} %GIDa_778518f3_3d70_4d5f_997f_17df4302258d  Port=5
  Adc0ScanGroup2Ref0 : Inport  RequirementInfo={} %GIDa_4d51d9ac_68cd_474e_b511_5bbbc9264d7b  Port=6
  Adc0ScanGroup2Ref1 : Inport  RequirementInfo={} %GIDa_f8618099_7dc5_498a_97eb_bfbda85dffb1  Port=7
  Adc0 Scan Group Strt and End Ref Voltage Diagc : Subsystem  RequirementInfo="{'linktype_rmi_doors' '000079f2 (/ESG Group/FDD Module Requirements/EA4 Specific/CM340A_AdcDiagc)' '#CM340A_204' 'true' 'REQ:  CM340A_204' '' } %GIDa_42a8a50a_2387_4959_8004_357af6557f2b"  Priority=20
      settings: AttributesFormatString=Priority = %<Priority>
  Bitwise Operator2 : simulink/Logic and Bit Operations/Bitwise Operator  logicop=OR  UseBitMask=off  NumInputPorts=2  BitMask=bin2dec('11011001')  BitMaskRealWorld=Stored Integer
  CopyRight2 : Subsystem  Description=|  mask(Copyright Information){none=on}
      | Copyright info block.                                               
      |                                                                     
      | Place copyright information at the top of every subsystem in design.
      mask prompts: none "No parameters"
      mask help: Place copyright information at the top of every subsystem in design.
      mask Display:
      | NxtrConf = 'Nexteer Confidential';
      | 
      | sys = bdroot; %handle for the current model ("system")
      | first = get_param(sys,'Created');
      | first = first(end-3:end);  %year is last four digits
      | 
      | last = get_param(sys,'LastModifiedDate');
      | if isempty(last)
      |     last = datestr(now,'yyyy');
      | else
      |     last = last(end-3:end);
      | end
      | 
      | if strcmp(first,last)
      |     fprintf('%s -- Copyright %s Nexteer',NxtrConf,first)
      | else
      |     fprintf('%s -- %s%s- %s Nexteer',NxtrConf,char(169),first,last)
      | end
  Data Store Read : DataStoreRead  DataStoreName=AdcDiagcSt
  Merge : Merge
  "State 0, 2, 4, 6" : Subsystem  TreatAsAtomicUnit=on
  State 1,3,5,7 : Subsystem  TreatAsAtomicUnit=on
  State Based Determination : SwitchCase  CaseConditions={[0,2,4,6]}
  Adc0 ParmByte : Outport
  wires:
  Adc0SelfDiag0/1 -> "State 0, 2, 4, 6"/1(Adc0SelfDiag0)
  Adc0SelfDiag2/1 -> "State 0, 2, 4, 6"/2(Adc0SelfDiag2)
  Adc0SelfDiag4/1 -> "State 0, 2, 4, 6"/3(Adc0SelfDiag4)
  Data Store Read/1 -> "State 0, 2, 4, 6"/4(Adc0DiagSt), State Based Determination/1
  State Based Determination/1 -> "State 0, 2, 4, 6"/Action
  State Based Determination/2 -> State 1,3,5,7/Action
  Adc0ScanGroup3Ref0/1 -> Adc0 Scan Group Strt and End Ref Voltage Diagc/1(Adc0ScanGroup3Ref0)
  Adc0ScanGroup3Ref1/1 -> Adc0 Scan Group Strt and End Ref Voltage Diagc/2(Adc0ScanGroup3Ref1)
  Adc0ScanGroup2Ref0/1 -> Adc0 Scan Group Strt and End Ref Voltage Diagc/3(Adc0ScanGroup2Ref0)
  Adc0ScanGroup2Ref1/1 -> Adc0 Scan Group Strt and End Ref Voltage Diagc/4(Adc0ScanGroup2Ref1)
  "State 0, 2, 4, 6"/1(Parameter Byte) -> Merge/1
  State 1,3,5,7/1(Parameter Byte) -> Merge/2
  Merge/1 -> Bitwise Operator2/1
  Adc0 Scan Group Strt and End Ref Voltage Diagc/1(Parameter Byte) -> Bitwise Operator2/2
  Bitwise Operator2/1 -> Adc0 ParmByte/1

== system CM340A_AdcDiagc/AdcDiagc/AdcDiagcPer1/Adc1 Diagc ==
  Adc1SelfDiag0 : Inport  RequirementInfo={} %GIDa_fcdc76d8_e1ba_4cde_9c3f_fc200b11d0f3
  Adc1SelfDiag2 : Inport  RequirementInfo={} %GIDa_f299f2ae_d981_419b_9259_89873c8e724e  Port=2
  Adc1SelfDiag4 : Inport  RequirementInfo={} %GIDa_bdbfccea_5048_4270_add7_62610089fb6d  Port=3
  Adc1ScanGroup3Ref0 : Inport  RequirementInfo={} %GIDa_53582631_2163_4437_beca_6b1c7064d2ac  Port=4
  Adc1ScanGroup3Ref1 : Inport  RequirementInfo={} %GIDa_f7c97e24_503f_4407_bd2e_c30d0aea58d8  Port=5
  Adc1ScanGroup2Ref0 : Inport  RequirementInfo={} %GIDa_460d229d_ce83_45dd_9f73_1d1a8299ca41  Port=6
  Adc1ScanGroup2Ref1 : Inport  RequirementInfo={} %GIDa_43678493_3608_4414_9b39_94d8cd4d0b6a  Port=7
  Adc1 Scan Group Strt and End Ref Voltage Diagc : Subsystem  RequirementInfo="{'linktype_rmi_doors' '000079f2 (/ESG Group/FDD Module Requirements/EA4 Specific/CM340A_AdcDiagc)' '#CM340A_204' 'true' 'REQ:  CM340A_204' '' } %GIDa_982bbfd4_d8b4_47b8_aecc_f635f4da0a89"  Priority=20
      settings: AttributesFormatString=Priority = %<Priority>
  Bitwise Operator : simulink/Logic and Bit Operations/Bitwise Operator  logicop=OR  UseBitMask=off  NumInputPorts=2  BitMask=bin2dec('11011001')  BitMaskRealWorld=Stored Integer
  CopyRight2 : Subsystem  Description=|  mask(Copyright Information){none=on}
      | Copyright info block.                                               
      |                                                                     
      | Place copyright information at the top of every subsystem in design.
      mask prompts: none "No parameters"
      mask help: Place copyright information at the top of every subsystem in design.
      mask Display:
      | NxtrConf = 'Nexteer Confidential';
      | 
      | sys = bdroot; %handle for the current model ("system")
      | first = get_param(sys,'Created');
      | first = first(end-3:end);  %year is last four digits
      | 
      | last = get_param(sys,'LastModifiedDate');
      | if isempty(last)
      |     last = datestr(now,'yyyy');
      | else
      |     last = last(end-3:end);
      | end
      | 
      | if strcmp(first,last)
      |     fprintf('%s -- Copyright %s Nexteer',NxtrConf,first)
      | else
      |     fprintf('%s -- %s%s- %s Nexteer',NxtrConf,char(169),first,last)
      | end
  Data Store Read : DataStoreRead  DataStoreName=AdcDiagcSt
  Merge : Merge
  State 0,2,4,6 : Subsystem  TreatAsAtomicUnit=on
  State 1,3,5,7 : Subsystem  TreatAsAtomicUnit=on
  State Based Determination : SwitchCase  CaseConditions={[0,2,4,6]}
  Adc1 ParmByte : Outport
  wires:
  Data Store Read/1 -> State 0,2,4,6/4(Adc1DiagSt), State Based Determination/1
  State Based Determination/2 -> State 1,3,5,7/Action
  State Based Determination/1 -> State 0,2,4,6/Action
  Adc1SelfDiag0/1 -> State 0,2,4,6/1(Adc1SelfDiag0)
  Adc1SelfDiag2/1 -> State 0,2,4,6/2(Adc1SelfDiag2)
  Adc1SelfDiag4/1 -> State 0,2,4,6/3(Adc1SelfDiag4)
  Adc1ScanGroup3Ref0/1 -> Adc1 Scan Group Strt and End Ref Voltage Diagc/1(Adc1ScanGroup3Ref0)
  Adc1ScanGroup3Ref1/1 -> Adc1 Scan Group Strt and End Ref Voltage Diagc/2(Adc1ScanGroup3Ref1)
  Adc1ScanGroup2Ref0/1 -> Adc1 Scan Group Strt and End Ref Voltage Diagc/3(Adc1ScanGroup2Ref0)
  Adc1ScanGroup2Ref1/1 -> Adc1 Scan Group Strt and End Ref Voltage Diagc/4(Adc1ScanGroup2Ref1)
  State 0,2,4,6/1(Parameter Byte) -> Merge/1
  State 1,3,5,7/1(Parameter Byte) -> Merge/2
  Merge/1 -> Bitwise Operator/1
  Adc1 Scan Group Strt and End Ref Voltage Diagc/1(Parameter Byte) -> Bitwise Operator/2
  Bitwise Operator/1 -> Adc1 ParmByte/1

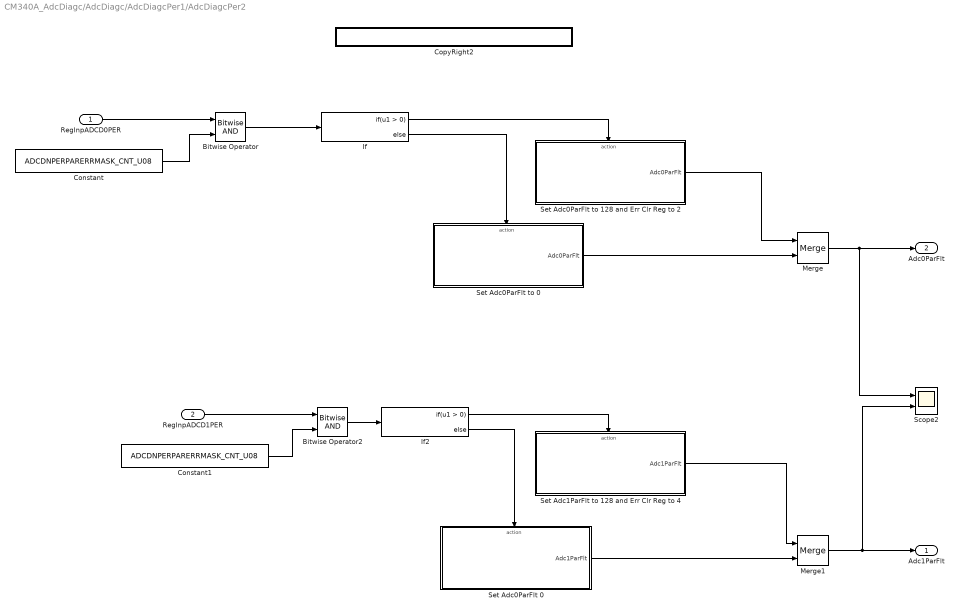
== system CM340A_AdcDiagc/AdcDiagc/AdcDiagcPer1/AdcDiagcPer2 ==
  RegInpADCD0PER : Inport
  RegInpADCD1PER : Inport  Port=2
  Bitwise Operator : simulink/Logic and Bit Operations/Bitwise Operator  logicop=AND  UseBitMask=off  NumInputPorts=2  BitMask=bin2dec('10000000')  BitMaskRealWorld=Stored Integer
  Bitwise Operator2 : simulink/Logic and Bit Operations/Bitwise Operator  logicop=AND  UseBitMask=off  NumInputPorts=2  BitMask=bin2dec('10000000')  BitMaskRealWorld=Stored Integer
  Constant : Constant  Value=ADCDNPERPARERRMASK_CNT_U08  OutDataTypeStr=uint8
  Constant1 : Constant  Value=ADCDNPERPARERRMASK_CNT_U08  OutDataTypeStr=uint8
  CopyRight2 : Subsystem  Description=|  mask(Copyright Information){none=on}
      | Copyright info block.                                               
      |                                                                     
      | Place copyright information at the top of every subsystem in design.
      mask prompts: none "No parameters"
      mask help: Place copyright information at the top of every subsystem in design.
      mask Display:
      | NxtrConf = 'Nexteer Confidential';
      | 
      | sys = bdroot; %handle for the current model ("system")
      | first = get_param(sys,'Created');
      | first = first(end-3:end);  %year is last four digits
      | 
      | last = get_param(sys,'LastModifiedDate');
      | if isempty(last)
      |     last = datestr(now,'yyyy');
      | else
      |     last = last(end-3:end);
      | end
      | 
      | if strcmp(first,last)
      |     fprintf('%s -- Copyright %s Nexteer',NxtrConf,first)
      | else
      |     fprintf('%s -- %s%s- %s Nexteer',NxtrConf,char(169),first,last)
      | end
  If : If
  If2 : If
  Merge : Merge
  Merge1 : Merge
  Scope2 : Scope  NumInputPorts=2
      settings: YMin=-5~-5  YMax=5~5  SaveName=ScopeData11
  Set Adc0ParFlt 0 : Subsystem  RequirementInfo="{'linktype_rmi_doors' '000079f2 (/ESG Group/FDD Module Requirements/EA4 Specific/CM340A_AdcDiagc)' '#CM340A_211' 'true' 'REQ:  CM340A_211' '' } %GIDa_f621ba00_abfa_4b34_9d45_2889bd17cb41"  TreatAsAtomicUnit=on
  Set Adc0ParFlt to 0 : Subsystem  RequirementInfo="{'linktype_rmi_doors' '000079f2 (/ESG Group/FDD Module Requirements/EA4 Specific/CM340A_AdcDiagc)' '#CM340A_211' 'true' 'REQ:  CM340A_211' '' } %GIDa_02eeba5e_fea9_4b04_89bb_99aa87e4bf35"  TreatAsAtomicUnit=on
  Set Adc0ParFlt to 128 and Err Clr Reg to 2 : Subsystem  RequirementInfo="{'linktype_rmi_doors' '000079f2 (/ESG Group/FDD Module Requirements/EA4 Specific/CM340A_AdcDiagc)' '#CM340A_211' 'true' 'REQ:  CM340A_211' '' } %GIDa_13bd7b1b_c35e_4ee8_bef0_a88e9046e5a7"  TreatAsAtomicUnit=on
  Set Adc1ParFlt to 128 and Err Clr Reg to 4 : Subsystem  RequirementInfo="{'linktype_rmi_doors' '000079f2 (/ESG Group/FDD Module Requirements/EA4 Specific/CM340A_AdcDiagc)' '#CM340A_211' 'true' 'REQ:  CM340A_211' '' } %GIDa_dd56c30d_d074_44b7_a42c_f1727676819c"  TreatAsAtomicUnit=on
  Adc1ParFlt : Outport
  Adc0ParFlt : Outport  Port=2
  wires:
  RegInpADCD0PER/1 -> Bitwise Operator/1
  Bitwise Operator/1 -> If/1
  Bitwise Operator2/1 -> If2/1
  Constant/1 -> Bitwise Operator/2
  Constant1/1 -> Bitwise Operator2/2
  If/1 -> Set Adc0ParFlt to 128 and Err Clr Reg to 2/Action
  If/2 -> Set Adc0ParFlt to 0/Action
  Set Adc0ParFlt to 128 and Err Clr Reg to 2/1(Adc0ParFlt) -> Merge/1
  Set Adc0ParFlt to 0/1(Adc0ParFlt) -> Merge/2
  RegInpADCD1PER/1 -> Bitwise Operator2/1
  Set Adc1ParFlt to 128 and Err Clr Reg to 4/1(Adc1ParFlt) -> Merge1/1
  Set Adc0ParFlt 0/1(Adc1ParFlt) -> Merge1/2
  If2/1 -> Set Adc1ParFlt to 128 and Err Clr Reg to 4/Action
  If2/2 -> Set Adc0ParFlt 0/Action
  Merge1/1 -> Scope2/2, Adc1ParFlt/1
  Merge/1 -> Scope2/1, Adc0ParFlt/1

== system CM340A_AdcDiagc/AdcDiagc/AdcDiagcPer1/CopyRight2 ==

== system CM340A_AdcDiagc/AdcDiagc/AdcDiagcPer1/NTC Fault Processing0 ==
  Adc0 ParmByte : Inport
  Adc0ParFlt : Inport  Port=2
  Add : Sum
  Atomic Subsystem : Subsystem  RequirementInfo="{'linktype_rmi_doors' '000079f2 (/ESG Group/FDD Module Requirements/EA4 Specific/CM340A_AdcDiagc)' '#CM340A_28' 'true' 'REQ:  CM340A_28' '' ; 'linktype_rmi_doors' '000079f2 (/ESG Group/FDD Module Requirements/EA4 Specific/CM340A_AdcDiagc)' '#CM340A_31' 'true' 'REQ:  CM340A_31' '' } %GIDa_f1ee7540_0919_4861_8305_ebbb47afc10d"  TreatAsAtomicUnit=on
  Constant3 : Constant  Value=Adc0Diagc
  CopyRight2 : Subsystem  Description=|  mask(Copyright Information){none=on}
      | Copyright info block.                                               
      |                                                                     
      | Place copyright information at the top of every subsystem in design.
      mask prompts: none "No parameters"
      mask help: Place copyright information at the top of every subsystem in design.
      mask Display:
      | NxtrConf = 'Nexteer Confidential';
      | 
      | sys = bdroot; %handle for the current model ("system")
      | first = get_param(sys,'Created');
      | first = first(end-3:end);  %year is last four digits
      | 
      | last = get_param(sys,'LastModifiedDate');
      | if isempty(last)
      |     last = datestr(now,'yyyy');
      | else
      |     last = last(end-3:end);
      | end
      | 
      | if strcmp(first,last)
      |     fprintf('%s -- Copyright %s Nexteer',NxtrConf,first)
      | else
      |     fprintf('%s -- %s%s- %s Nexteer',NxtrConf,char(169),first,last)
      | end
  Data Type Conversion : DataTypeConversion  OutDataTypeStr=Enum: SigQlfr1
  Enumerated Constant : simulink/Sources/Enumerated Constant  OutDataTypeStr=Enum: SigQlfr1  Value=SigQlfr1.SIGQLFR_FAILD  SampleTime=inf
  GetNtcQlfr : Subsystem  RequirementInfo={} %GIDa_aac3a6f9_1ce1_44c6_a21e_d7cfd00595b5
  Relational Operator : RelationalOperator  Operator===  OutDataTypeStr=boolean
  SetNtcSts : Subsystem  RequirementInfo="{'linktype_rmi_doors' '000079f2 (/ESG Group/FDD Module Requirements/EA4 Specific/CM340A_AdcDiagc)' '#CM340A_22' 'true' 'REQ:  CM340A_22' '' } %GIDa_895c4299_af49_4ccd_8f8d_942893b281fe"
  Adc0Faild : Outport
  wires:
  Constant3/1 -> SetNtcSts/1(NtcNr), GetNtcQlfr/1(NtcNr)  "NtcNr"
  Atomic Subsystem/1(NtcSts) -> SetNtcSts/3(NtcSts)
  Atomic Subsystem/2(DebStep) -> SetNtcSts/4(DebStep)
  Adc0 ParmByte/1 -> Add/1
  GetNtcQlfr/1(NtcQlfr) -> Data Type Conversion/1
  Data Type Conversion/1 -> Relational Operator/1
  Enumerated Constant/1 -> Relational Operator/2
  Relational Operator/1 -> Adc0Faild/1
  Add/1 -> SetNtcSts/2(NtcStInfo), Atomic Subsystem/1(NtcStInfo)
  Adc0ParFlt/1 -> Add/2
